simulink library "cyclopsLib"  (R2020a)
settings: Solver=VariableStepAuto  StartTime=0.0  StopTime=10.0  RelTol=1e-3
values from neighbouring files (symbols this model uses):
  agc_delay_lag = 32    [rev0BB_setup.m]
  agc_detector_coef = ones(1,agc_detector_taps)./agc_detector_taps    [rev0BB_setup.m]
  agc_sat_low = -agcSaturation    (= -12)    [rev0BB_setup.m]
  agc_sat_up = agcSaturation    (= 12)    [rev0BB_setup.m]
  agcDesired = 0    [rev0BB_setup.m]
  agcExpDomain = agcSaturation    (= 12)    [rev0BB_setup.m]
  agcExpResolution = 2^-3    (= 0.125)    [rev0BB_setup.m]
  agcPwrAvgNum = 128    [rev0BB_setup.m]
  agcSettleThresh = 0.65    [rev0BB_setup.m]
  agcStep = 2^-8    (= 0.00390625)    [rev0BB_setup.m]
  atanDomain = 5    [rev0BB_setup.m]
  atanResolution = 2^-9    (= 0.001953125)    [rev0BB_setup.m]
  bitsPerSymbolHeader = log2(radixHeader)    [rev0BB_setup.m]
  bitsPerSymbolMax = log2(radixMax)    [rev0BB_setup.m]
  cefEarlyWarning = 256    [rev0BB_setup.m]
  cefLen = length(x_CEF)    [rev0BB_setup.m]
  coarseCFOAdaptDelay = 1    [rev0BB_setup.m]
  cr_i = 0.020    (= 0.02)    [rev0BB_setup.m]
  cr_i_preamp = 2^-9    (= 0.001953125)    [rev0BB_setup.m]
  cr_int1_sat_low = -cr_integrator1_saturation    (= -0.6)    [rev0BB_setup.m]
  cr_int1_sat_up = cr_integrator1_saturation    (= 0.6)    [rev0BB_setup.m]
  cr_integrator1_decay = 1    [rev0BB_setup.m]
  cr_integrator1_saturation = 0.6    [rev0BB_setup.m]
  cr_mult_pipeline = 1    [rev0BB_setup.m]
  cr_p = 0.015    [rev0BB_setup.m]
  cr_sat2_low = -cr_saturation2    (= -0.6)    [rev0BB_setup.m]
  cr_sat2_up = cr_saturation2    (= 0.6)    [rev0BB_setup.m]
  cr_smooth_num = (1/cr_smooth_samples).*ones(1, cr_smooth_samples)    [rev0BB_setup.m]
  D_32 = [ 1,  4,  8,  2, 16]    [golay.m]    (also in rev0BB_setup.m)
  dataLenSymbols = header_len_bytes*8/bitsPerSymbolHeader + frame_len_bytes*8/bitsPerSymbol    [rev0BB_setup.m]
  delayToOutputFromDataFSM = lmsEqDepth/2-1 + regular_pipeline*9 + cr_mult_pipeline*4    (= 31)    [rev0BB_setup.m]
  enableTRFreqCorrection = true    [rev0BB_setup.m]
  expDomain = 3.3    [rev0BB_setup.m]
  expResolution = 2^-5    (= 0.03125)    [rev0BB_setup.m]
  expTol = .1    (= 0.1)    [rev0BB_setup.m]
  forceSlowRxStrobed = false    [rev0BB_setup.m]
  frac_lut_domain_cr = 64    [rev0BB_setup.m]
  frac_lut_range_max_coarse_cfo = 127    [rev0BB_setup.m]
  frac_lut_range_max_cr = 127    [rev0BB_setup.m]
  frac_lut_range_min_coarse_cfo = -frac_lut_range_max_coarse_cfo    (= -127)    [rev0BB_setup.m]
  frac_lut_range_min_cr = -frac_lut_range_max_cr    (= -127)    [rev0BB_setup.m]
  frac_lut_table_breaks_coarse_cfo = -frac_lut_domain_coarse_cfo:frac_lut_res_coarse_cfo:(frac_lut_domain_coarse_cfo-1)    [rev0BB_setup.m]
  frac_lut_table_breaks_cr = -frac_lut_domain_cr:frac_lut_res_cr:(frac_lut_domain_cr-1)    [rev0BB_setup.m]
  frac_lut_table_data_coarse_cfo = 1./frac_lut_table_breaks_coarse_cfo    [rev0BB_setup.m]
  frac_lut_table_data_cr = 1./frac_lut_table_breaks_cr    [rev0BB_setup.m]
  golay_type = 32    [rev0BB_setup.m]
  header_len_bytes = 8    [rev0BB_setup.m]
  lmsEqDepth = 38    [rev0BB_setup.m]
  lmsStep_init = 0.012    [rev0BB_setup.m]
  lmsStep_meta = (lmsStep_final - lmsStep_init)/cefLen    [rev0BB_setup.m]
  lnDomain = 16    [rev0BB_setup.m]
  lnResolution = 2^-3    (= 0.125)    [rev0BB_setup.m]
  minSTFPeaks = 3    [rev0BB_setup.m]
  mod_scheme_len_bytes = 1    [rev0BB_setup.m]
  modBPS = [1, 2, 4]    [rev0BB_setup.m]
  modKeys = [0, 1, 2]    [rev0BB_setup.m]
  mult_pipeline = 1    [rev0BB_setup.m]
  overSample = 4    [berCurve.m]    (also in rev0BB_setup.m)
  overSamplePer = 1/overSampleFreq    (= 1.25e-08)    [rev0BB_setup.m]
  qam16_demod_scale_factor = qam16_hdl_distance/qam16_power_normalized_distance    [rev0BB_setup.m]
  rcRxFilt = rcSqrtFilt    [rev0BB_setup.m]
  rcTxFilt = rcSqrtFilt    [rev0BB_setup.m]
  regular_pipeline = 1    [rev0BB_setup.m]
  rx_gain = 1    [rev0BB_setup.m]
  rx_gain_i = 1    [rev0BB_setup.m]
  rx_gain_q = 1    [rev0BB_setup.m]
  RxFeedbackPipelining = 128*3    (= 384)    [rev0BB_setup.m]
  stfLen = length(x_STF)    [rev0BB_setup.m]
  timing_differentiator_grpDelay_roundUp = ceil((timing_differentiator_len)/2)    [rev0BB_setup.m]
  timing_integrator1_decay = 0.999    [rev0BB_setup.m]
  timing_p = -1/2^2 -1/2^3    (= -0.375)    [rev0BB_setup.m]
  timing_tolerance = 4    [rev0BB_setup.m]
  timingRecoveryDoneSamplesEarly = 1    [rev0BB_setup.m]
  timingRecoveryDoneSamplesEarlyExtraDelay = -timingRecoveryDoneSamplesEarly+1    (= 0)    [rev0BB_setup.m]
  tr_int1_sat_low = -timing_integrate1_saturate    (= -0.0025)    [rev0BB_setup.m]
  tr_int1_sat_up = timing_integrate1_saturate    (= 0.0025)    [rev0BB_setup.m]
  tr_sat2_low = -timing_saturate2    (= -0.005)    [rev0BB_setup.m]
  tr_sat2_up = timing_saturate2    (= 0.005)    [rev0BB_setup.m]
  trigger = 0.40    (= 0.4)    [rev0BB_setup.m]
  trigger_tolerance = 0.35    [rev0BB_setup.m]
  W_32 = [-1,  1, -1,  1, -1]    [golay.m]    (also in rev0BB_setup.m)
  x_STFRepCount = nSpectrum_STFRepCount_short    (= 60)    [rev0BB_setup.m]
undefined symbols (not defined in the file or in its folder): agc_on, cr_integrator2_saturation, Fast_Rx_Partition, Fast_Slim_Rx_Partition, Feedback_Pipeline, freeze_en_agc, freeze_en_cr_int1, freeze_en_cr_int2, freeze_en_cr_phase, freeze_en_tr_int1, freeze_en_tr_int2, freeze_en_tr_phase, freeze_on_cef_done, freeze_on_stf_done, freeze_on_valid, i, post_cr_i_offset, post_cr_q_offset, rx_offset_correction_i, rx_offset_correction_q, Slow_Rx_Partition, timing_i, timing_i_pre_scale
libraries: simulink x62, helperLib x48, golayLib x15, commdigbbndpm3 x8, commdigbbndam3 x4, commfilt2 x3, hdlsllib x2, dspfdesign x1, simulink_need_slupdate x1, dspsigops x1, dsphdlsigops x1, $bdroot x1
(part 1 of 5)
settings Model: Creator=cyarp  LastModifiedBy=cyarp

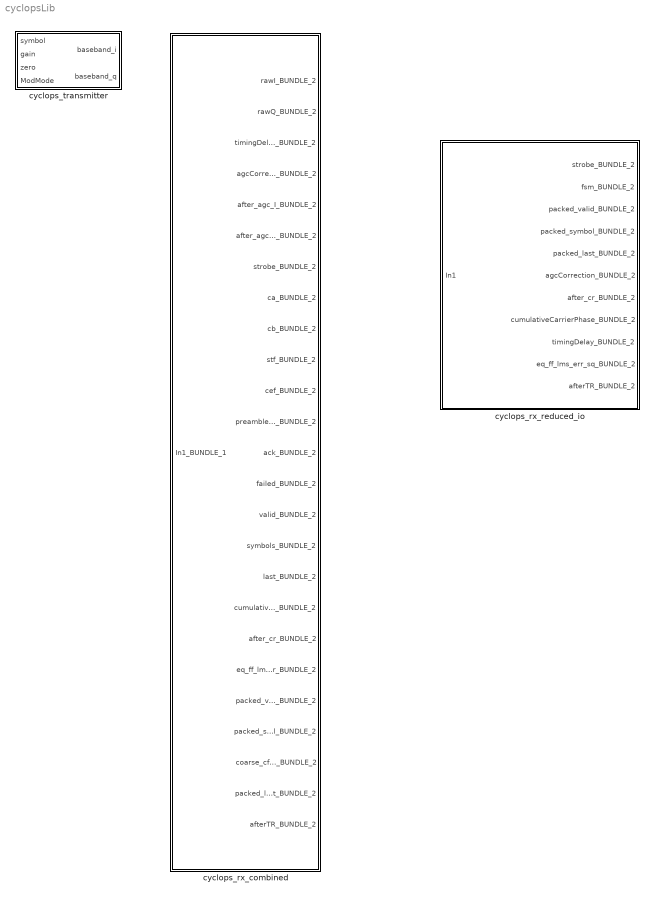
== system cyclopsLib ==
  cyclops_rx_combined : Subsystem  mask(Cyclops Rx){Fast_Slim_Rx_Partition=Fast_Slim_Rx_Partition, Fast_Rx_Partition=Fast_Rx_Partition, Slow_Rx_Partition=Slow_Rx_Partition, Feedback_Pipeline=Feedback_Pipeline}
      mask help: The Cyclops Rx with parameters for partitioning
  cyclops_rx_reduced_io : Subsystem  mask(Cyclops Rx (Reduced I/O)){Fast_Slim_Rx_Partition=1, Fast_Rx_Partition=2, Slow_Rx_Partition=2, Feedback_Pipeline=RxFeedbackPipelining}
      mask help: The Cyclops Rx with parameters for partitioning and reduced I/O
  cyclops_transmitter : Subsystem  mask(Cyclops Transmitter){Tx_Partition=1}
      mask help: The single channel transmitter for Cyclops. Parameterized with partition numbers

== system cyclopsLib/cyclops_rx_combined ==
  note: This feedback delay path is not latency critical.
      | Further pripelining should be OK
  In1_BUNDLE_1 : Inport
  fast_rx : Subsystem  TreatAsAtomicUnit=on
  slow_rx_encapsulated : Subsystem
  rawI_BUNDLE_2 : Outport  VectorParamsAs1DForOutWhenUnconnected=off
  rawQ_BUNDLE_2 : Outport  Port=2  VectorParamsAs1DForOutWhenUnconnected=off
  timingDelay_BUNDLE_2 : Outport  Port=3  VectorParamsAs1DForOutWhenUnconnected=off
  agcCorrection_BUNDLE_2 : Outport  Port=4  VectorParamsAs1DForOutWhenUnconnected=off
  after_agc_I_BUNDLE_2 : Outport  Port=5  VectorParamsAs1DForOutWhenUnconnected=off
  after_agc_Q_BUNDLE_2 : Outport  Port=6  VectorParamsAs1DForOutWhenUnconnected=off
  strobe_BUNDLE_2 : Outport  Port=7  VectorParamsAs1DForOutWhenUnconnected=off
  ca_BUNDLE_2 : Outport  Port=8  VectorParamsAs1DForOutWhenUnconnected=off
  cb_BUNDLE_2 : Outport  Port=9  VectorParamsAs1DForOutWhenUnconnected=off
  stf_BUNDLE_2 : Outport  Port=10  VectorParamsAs1DForOutWhenUnconnected=off
  cef_BUNDLE_2 : Outport  Port=11  VectorParamsAs1DForOutWhenUnconnected=off
  preambleDone_upsample_BUNDLE_2 : Outport  Port=12  VectorParamsAs1DForOutWhenUnconnected=off
  ack_BUNDLE_2 : Outport  Port=13  VectorParamsAs1DForOutWhenUnconnected=off
  failed_BUNDLE_2 : Outport  Port=14  VectorParamsAs1DForOutWhenUnconnected=off
  valid_BUNDLE_2 : Outport  Port=15  VectorParamsAs1DForOutWhenUnconnected=off
  symbols_BUNDLE_2 : Outport  Port=16  VectorParamsAs1DForOutWhenUnconnected=off
  last_BUNDLE_2 : Outport  Port=17  VectorParamsAs1DForOutWhenUnconnected=off
  cumulativeCarrierPhase_BUNDLE_2 : Outport  Port=18  VectorParamsAs1DForOutWhenUnconnected=off
  after_cr_BUNDLE_2 : Outport  Port=19  VectorParamsAs1DForOutWhenUnconnected=off
  eq_ff_lms_err_BUNDLE_2 : Outport  Port=20  VectorParamsAs1DForOutWhenUnconnected=off
  packed_valid_BUNDLE_2 : Outport  Port=21  VectorParamsAs1DForOutWhenUnconnected=off
  packed_symbol_BUNDLE_2 : Outport  Port=22  VectorParamsAs1DForOutWhenUnconnected=off
  coarse_cfo_correct_steps_BUNDLE_2 : Outport  Port=23  VectorParamsAs1DForOutWhenUnconnected=off
  packed_last_BUNDLE_2 : Outport  Port=24  VectorParamsAs1DForOutWhenUnconnected=off
  afterTR_BUNDLE_2 : Outport  Port=25
  wires:
  slow_rx_encapsulated/21(afterTR) -> afterTR_BUNDLE_2/1
  slow_rx_encapsulated/20(packet_reset_feedback) -> fast_rx/3(packet_reset_feedback)
  In1_BUNDLE_1/1 -> fast_rx/1(In1)
  fast_rx/4(rawI) -> rawI_BUNDLE_2/1
  fast_rx/5(rawQ) -> rawQ_BUNDLE_2/1
  fast_rx/6(timingDelay) -> timingDelay_BUNDLE_2/1
  fast_rx/7(agcCorrection) -> agcCorrection_BUNDLE_2/1
  fast_rx/8(after_agc_I) -> after_agc_I_BUNDLE_2/1
  fast_rx/9(after_agc_Q) -> after_agc_Q_BUNDLE_2/1
  fast_rx/1(data_out) -> slow_rx_encapsulated/1(data_in)
  fast_rx/2(agcPwrEst) -> slow_rx_encapsulated/2(agc_pwr_est)
  fast_rx/3(push) -> slow_rx_encapsulated/3(enb)
  slow_rx_encapsulated/1(strobe) -> strobe_BUNDLE_2/1
  slow_rx_encapsulated/2(ca) -> ca_BUNDLE_2/1
  slow_rx_encapsulated/3(cb) -> cb_BUNDLE_2/1
  slow_rx_encapsulated/4(stf) -> stf_BUNDLE_2/1
  slow_rx_encapsulated/5(cef) -> cef_BUNDLE_2/1
  slow_rx_encapsulated/6(preambleDone_upsample) -> preambleDone_upsample_BUNDLE_2/1
  slow_rx_encapsulated/7(ack) -> ack_BUNDLE_2/1
  slow_rx_encapsulated/8(failed) -> failed_BUNDLE_2/1
  slow_rx_encapsulated/9(valid) -> valid_BUNDLE_2/1
  slow_rx_encapsulated/10(symbols) -> symbols_BUNDLE_2/1
  slow_rx_encapsulated/11(last) -> last_BUNDLE_2/1
  slow_rx_encapsulated/12(cumulativeCarrierPhase) -> cumulativeCarrierPhase_BUNDLE_2/1
  slow_rx_encapsulated/13(after_cr) -> after_cr_BUNDLE_2/1
  slow_rx_encapsulated/14(eq_ff_lms_err) -> eq_ff_lms_err_BUNDLE_2/1
  slow_rx_encapsulated/15(freeze_out_pipelined) -> fast_rx/2(freeze)
  slow_rx_encapsulated/16(packed_valid) -> packed_valid_BUNDLE_2/1
  slow_rx_encapsulated/17(packed_symbol) -> packed_symbol_BUNDLE_2/1
  slow_rx_encapsulated/18(coarse_cfo_correct_steps) -> coarse_cfo_correct_steps_BUNDLE_2/1
  slow_rx_encapsulated/19(packed_last) -> packed_last_BUNDLE_2/1

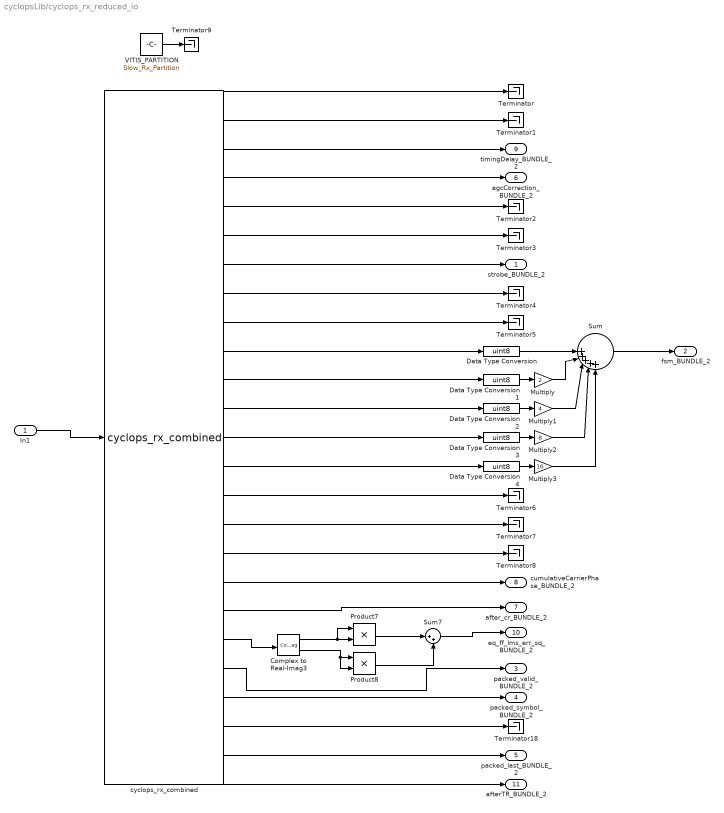
== system cyclopsLib/cyclops_rx_reduced_io ==
  In1 : Inport
  Complex to Real-Imag3 : ComplexToRealImag
  Data Type Conversion{,1..4} (5 alike) : DataTypeConversion  OutDataTypeStr=uint8
  Multiply : Gain  Gain=2  OutDataTypeStr=Inherit: Same as input
  Multiply1 : Gain  Gain=4  OutDataTypeStr=Inherit: Same as input
  Multiply2 : Gain  Gain=8  OutDataTypeStr=Inherit: Same as input
  Multiply3 : Gain  Gain=16  ParamDataTypeStr=Inherit: Same as input
  Product7 : Product
  Product8 : Product
  Sum : Sum  Inputs=||||+++++  OutDataTypeStr=Inherit: Same as first input
  Sum7 : Sum  Inputs=|++
  Terminator{,1..9,18} (11 alike) : Terminator
  VITIS_PARTITION : Constant  Value=Slow_Rx_Partition
  cyclops_rx_combined : $bdroot/cyclops_rx_combined  Fast_Slim_Rx_Partition=Fast_Slim_Rx_Partition  Fast_Rx_Partition=Fast_Rx_Partition  Slow_Rx_Partition=Slow_Rx_Partition  Feedback_Pipeline=Feedback_Pipeline
  strobe_BUNDLE_2 : Outport
  fsm_BUNDLE_2 : Outport  Port=2
  packed_valid_BUNDLE_2 : Outport  Port=3
  packed_symbol_BUNDLE_2 : Outport  Port=4
  packed_last_BUNDLE_2 : Outport  Port=5
  agcCorrection_BUNDLE_2 : Outport  Port=6
  after_cr_BUNDLE_2 : Outport  Port=7
  cumulativeCarrierPhase_BUNDLE_2 : Outport  Port=8
  timingDelay_BUNDLE_2 : Outport  Port=9
  eq_ff_lms_err_sq_BUNDLE_2 : Outport  Port=10
  afterTR_BUNDLE_2 : Outport  Port=11
  wires:
  cyclops_rx_combined/25 -> afterTR_BUNDLE_2/1
  cyclops_rx_combined/18 -> cumulativeCarrierPhase_BUNDLE_2/1
  In1/1 -> cyclops_rx_combined/1
  cyclops_rx_combined/3 -> timingDelay_BUNDLE_2/1
  cyclops_rx_combined/24 -> packed_last_BUNDLE_2/1
  cyclops_rx_combined/9 -> Terminator5/1
  cyclops_rx_combined/12 -> Data Type Conversion2/1
  cyclops_rx_combined/5 -> Terminator2/1
  cyclops_rx_combined/21 -> packed_valid_BUNDLE_2/1
  Complex to Real-Imag3/1 -> Product7/1, Product7/2
  Data Type Conversion4/1 -> Multiply3/1
  cyclops_rx_combined/17 -> Terminator8/1
  cyclops_rx_combined/16 -> Terminator7/1
  cyclops_rx_combined/10 -> Data Type Conversion/1
  cyclops_rx_combined/14 -> Data Type Conversion4/1
  Multiply2/1 -> Sum/4
  cyclops_rx_combined/8 -> Terminator4/1
  cyclops_rx_combined/4 -> agcCorrection_BUNDLE_2/1
  Multiply3/1 -> Sum/5
  cyclops_rx_combined/23 -> Terminator18/1
  cyclops_rx_combined/19 -> after_cr_BUNDLE_2/1
  cyclops_rx_combined/2 -> Terminator1/1
  Sum7/1 -> eq_ff_lms_err_sq_BUNDLE_2/1
  Multiply1/1 -> Sum/3
  Product8/1 -> Sum7/2
  Data Type Conversion3/1 -> Multiply2/1
  Multiply/1 -> Sum/2
  Complex to Real-Imag3/2 -> Product8/2, Product8/1
  cyclops_rx_combined/11 -> Data Type Conversion1/1
  cyclops_rx_combined/6 -> Terminator3/1
  Sum/1 -> fsm_BUNDLE_2/1
  cyclops_rx_combined/13 -> Data Type Conversion3/1
  Product7/1 -> Sum7/1
  Data Type Conversion1/1 -> Multiply/1
  cyclops_rx_combined/20 -> Complex to Real-Imag3/1
  Data Type Conversion/1 -> Sum/1
  Data Type Conversion2/1 -> Multiply1/1
  cyclops_rx_combined/1 -> Terminator/1
  cyclops_rx_combined/15 -> Terminator6/1
  cyclops_rx_combined/7 -> strobe_BUNDLE_2/1
  cyclops_rx_combined/22 -> packed_symbol_BUNDLE_2/1
  VITIS_PARTITION/1 -> Terminator9/1

== system cyclopsLib/cyclops_transmitter ==
  note: Logic for zero filling in upsample
  symbol : Inport  SampleTime=overSamplePer
  gain : Inport  Port=2  SampleTime=overSamplePer
  zero : Inport  Port=3  OutDataTypeStr=boolean  SampleTime=overSamplePer
  ModMode : Inport  Port=4  SampleTime=overSamplePer
  Compare To Zero : simulink/Logic and Bit Operations/Compare To Zero  relop=~=  OutDataTypeStr=boolean
  Constant : Constant  Value=0  OutDataTypeStr=Inherit: Inherit via back propagation  SampleTime=-1
  Constant1 : Constant  Value=0  OutDataTypeStr=Inherit: Inherit via back propagation  SampleTime=-1
  Logical Operator : Logic  Operator=OR  AllPortsSameDT=off  OutDataTypeStr=boolean
  Real-Imag to Complex : RealImagToComplex
  Switch : Switch
  Terminator2 : Terminator
  VITIS_PARTITION : Constant  Value=Tx_Partition
  modulator : Subsystem
  part2_noLPF : Subsystem
  pipeline_delay1 : Delay  DelayLength=regular_pipeline
  raised_cosine : Subsystem
  zero_fill_counter : Subsystem
  baseband_i : Outport  SampleTime=overSamplePer  InitialOutput=[0]  VectorParamsAs1DForOutWhenUnconnected=off
  baseband_q : Outport  Port=2  SampleTime=overSamplePer  InitialOutput=[0]  VectorParamsAs1DForOutWhenUnconnected=off
  wires:
  pipeline_delay1/1 -> raised_cosine/1(In1)
  zero/1 -> Logical Operator/1
  Constant1/1 -> Real-Imag to Complex/2
  Constant/1 -> Real-Imag to Complex/1
  Real-Imag to Complex/1 -> Switch/1
  Logical Operator/1 -> Switch/2
  Compare To Zero/1 -> Logical Operator/2
  zero_fill_counter/1(Out1) -> Compare To Zero/1
  Switch/1 -> pipeline_delay1/1
  ModMode/1 -> modulator/1(mod_mode)
  symbol/1 -> modulator/2(symbol)
  modulator/1(point) -> Switch/3
  VITIS_PARTITION/1 -> Terminator2/1
  gain/1 -> part2_noLPF/1(Gain)
  raised_cosine/1(Out1) -> part2_noLPF/2(In)
  part2_noLPF/1(I) -> baseband_i/1
  part2_noLPF/2(Q) -> baseband_q/1

== system cyclopsLib/cyclops_rx_combined/fast_rx ==
  In1 : Inport
  freeze : Inport  Port=2
  packet_reset_feedback : Inport  Port=3
  fast_rx_baseband_encapsulated : Subsystem
  fast_rx_baseband_slim_encapsulated : Subsystem
  data_out : Outport  VectorParamsAs1DForOutWhenUnconnected=off
  agcPwrEst : Outport  Port=2  VectorParamsAs1DForOutWhenUnconnected=off
  push : Outport  Port=3  VectorParamsAs1DForOutWhenUnconnected=off
  rawI : Outport  Port=4  VectorParamsAs1DForOutWhenUnconnected=off
  rawQ : Outport  Port=5  VectorParamsAs1DForOutWhenUnconnected=off
  timingDelay : Outport  Port=6  VectorParamsAs1DForOutWhenUnconnected=off
  agcCorrection : Outport  Port=7  VectorParamsAs1DForOutWhenUnconnected=off
  after_agc_I : Outport  Port=8  VectorParamsAs1DForOutWhenUnconnected=off
  after_agc_Q : Outport  Port=9  VectorParamsAs1DForOutWhenUnconnected=off
  wires:
  packet_reset_feedback/1 -> fast_rx_baseband_encapsulated/3(packet_reset_feedback)
  freeze/1 -> fast_rx_baseband_slim_encapsulated/2(agc_freeze)
  fast_rx_baseband_slim_encapsulated/3(rawI) -> rawI/1
  fast_rx_baseband_slim_encapsulated/4(rawQ) -> rawQ/1
  fast_rx_baseband_slim_encapsulated/5(agcPwrEst) -> agcPwrEst/1
  fast_rx_baseband_slim_encapsulated/6(agcCorrection) -> agcCorrection/1
  fast_rx_baseband_encapsulated/2(data_out) -> data_out/1
  fast_rx_baseband_encapsulated/1(push) -> push/1
  fast_rx_baseband_encapsulated/5(after_agc_Q) -> after_agc_Q/1
  fast_rx_baseband_encapsulated/3(timing_delay) -> timingDelay/1
  fast_rx_baseband_encapsulated/4(after_agc_I) -> after_agc_I/1
  fast_rx_baseband_slim_encapsulated/1(sig_out_i) -> fast_rx_baseband_encapsulated/1(sig_in_i)
  fast_rx_baseband_slim_encapsulated/2(sig_out_q) -> fast_rx_baseband_encapsulated/2(sig_in_q)
  In1/1 -> fast_rx_baseband_slim_encapsulated/1(baseband_in)

== system cyclopsLib/cyclops_rx_combined/slow_rx_encapsulated ==
  note: This feedback delay path is not latency critical.
      | Further pripelining should be OK
  data_in : Inport
  agc_pwr_est : Inport  Port=2
  enb : Inport  Port=3
  Delay1 : Delay  Commented=on  DelayLength=128  InitialCondition=false
  Terminator : Terminator
  VITIS_PARTITION : Constant  Value=Slow_Rx_Partition
  slow_rx : Subsystem  TreatAsAtomicUnit=on
  strobe : Outport  VectorParamsAs1DForOutWhenUnconnected=off
  ca : Outport  Port=2  VectorParamsAs1DForOutWhenUnconnected=off
  cb : Outport  Port=3  VectorParamsAs1DForOutWhenUnconnected=off
  stf : Outport  Port=4  VectorParamsAs1DForOutWhenUnconnected=off
  cef : Outport  Port=5  VectorParamsAs1DForOutWhenUnconnected=off
  preambleDone_upsample : Outport  Port=6  VectorParamsAs1DForOutWhenUnconnected=off
  ack : Outport  Port=7  VectorParamsAs1DForOutWhenUnconnected=off
  failed : Outport  Port=8  VectorParamsAs1DForOutWhenUnconnected=off
  valid : Outport  Port=9  VectorParamsAs1DForOutWhenUnconnected=off
  symbols : Outport  Port=10  VectorParamsAs1DForOutWhenUnconnected=off
  last : Outport  Port=11  VectorParamsAs1DForOutWhenUnconnected=off
  cumulativeCarrierPhase : Outport  Port=12  VectorParamsAs1DForOutWhenUnconnected=off
  after_cr : Outport  Port=13  VectorParamsAs1DForOutWhenUnconnected=off
  eq_ff_lms_err : Outport  Port=14  VectorParamsAs1DForOutWhenUnconnected=off
  freeze_out_pipelined : Outport  Port=15  VectorParamsAs1DForOutWhenUnconnected=off
  packed_valid : Outport  Port=16  VectorParamsAs1DForOutWhenUnconnected=off
  packed_symbol : Outport  Port=17  VectorParamsAs1DForOutWhenUnconnected=off
  coarse_cfo_correct_steps : Outport  Port=18  VectorParamsAs1DForOutWhenUnconnected=off
  packed_last : Outport  Port=19  VectorParamsAs1DForOutWhenUnconnected=off
  packet_reset_feedback : Outport  Port=20
  afterTR : Outport  Port=21
  wires:
  slow_rx/21(afterTR) -> afterTR/1
  slow_rx/20(packet_reset_feedback) -> packet_reset_feedback/1
  slow_rx/11(last) -> last/1
  slow_rx/12(cumulativeCarrierPhase) -> cumulativeCarrierPhase/1
  slow_rx/8(failed) -> failed/1
  slow_rx/16(packed_symbol) -> packed_symbol/1
  slow_rx/15(packed_valid) -> packed_valid/1
  slow_rx/13(after_cr) -> after_cr/1
  slow_rx/14(eq_ff_lms_err) -> eq_ff_lms_err/1
  data_in/1 -> slow_rx/1(data_in)
  slow_rx/6(preambleDone_upsample) -> preambleDone_upsample/1
  agc_pwr_est/1 -> slow_rx/2(agc_pwr_est)
  enb/1 -> slow_rx/3(enb)
  slow_rx/1(strobe) -> strobe/1
  slow_rx/2(ca) -> ca/1
  slow_rx/3(cb) -> cb/1
  slow_rx/4(stf) -> stf/1
  slow_rx/5(cef) -> cef/1
  slow_rx/7(ack) -> ack/1
  slow_rx/10(symbols) -> symbols/1
  slow_rx/9(valid) -> valid/1
  VITIS_PARTITION/1 -> Terminator/1
  slow_rx/17(freeze_out) -> freeze_out_pipelined/1
  slow_rx/18(coarse_cfo_correct_steps) -> coarse_cfo_correct_steps/1
  slow_rx/19(packed_last) -> packed_last/1

== system cyclopsLib/cyclops_transmitter/modulator ==
  mod_mode : Inport
  symbol : Inport  Port=2
  BPSK Modulator Baseband : commdigbbndpm3/BPSK Modulator Baseband  Ph=0  outDtype=single  outWordLen=16  outUDDataType=sfix(16)  outFracLenMode=User-defined  outFracLen=13  outDataTypeStr=single  outLastDataTypeStr=single
  Bitwise Operator : simulink/Logic and Bit Operations/Bitwise Operator  logicop=AND  UseBitMask=off  NumInputPorts=2  BitMask=bin2dec('11011001')  BitMaskRealWorld=Stored Integer
  Bitwise Operator1 : simulink/Logic and Bit Operations/Bitwise Operator  logicop=AND  UseBitMask=off  NumInputPorts=2  BitMask=bin2dec('11011001')  BitMaskRealWorld=Stored Integer
  Bitwise Operator2 : simulink/Logic and Bit Operations/Bitwise Operator  logicop=AND  UseBitMask=off  NumInputPorts=2  BitMask=bin2dec('11011001')  BitMaskRealWorld=Stored Integer
  Constant : Constant  Value=bin2dec('000001')  OutDataTypeStr=Inherit: Inherit via back propagation
  Constant1 : Constant  Value=bin2dec('000011')  OutDataTypeStr=Inherit: Inherit via back propagation
  Constant2 : Constant  OutDataTypeStr=Inherit: Inherit via back propagation  SampleTime=-1
  Constant3 : Constant  Value=bin2dec('001111')  OutDataTypeStr=Inherit: Inherit via back propagation
  Data Type Conversion : DataTypeConversion  OutDataTypeStr=uint32
  Data Type Conversion1 : DataTypeConversion  OutDataTypeStr=uint32
  Data Type Conversion2 : DataTypeConversion  OutDataTypeStr=uint32
  Data Type Conversion3 : DataTypeConversion  Commented=on  OutDataTypeStr=fixdt(0,1,0)
  Data Type Conversion4 : DataTypeConversion  Commented=on  OutDataTypeStr=fixdt(0,2,0)
  Data Type Conversion5 : DataTypeConversion  Commented=on  OutDataTypeStr=fixdt(0,4,0)
  Extract Bits : simulink/Logic and Bit Operations/Extract Bits  Commented=on  bitsToExtract=Range of bits  numBits=8  bitIdxRange=[0 0]  outScalingMode=Preserve fixed-point scaling
  Extract Bits1 : simulink/Logic and Bit Operations/Extract Bits  Commented=on  bitsToExtract=Range of bits  numBits=8  bitIdxRange=[0 1]  outScalingMode=Preserve fixed-point scaling
  Extract Bits2 : simulink/Logic and Bit Operations/Extract Bits  Commented=on  bitsToExtract=Range of bits  numBits=8  bitIdxRange=[0 3]  outScalingMode=Preserve fixed-point scaling
  Multiport Switch : MultiPortSwitch
  QPSK Modulator Baseband : commdigbbndpm3/QPSK Modulator Baseband  InType=Integer  Enc=Gray  Ph=pi/4  outDtype=single  outWordLen=16  outUDDataType=sfix(16)  outFracLenMode=User-defined  outFracLen=13  outDataTypeStr=single  outLastDataTypeStr=single
  Rectangular QAM Modulator Baseband : commdigbbndam3/Rectangular QAM Modulator Baseband  M=16  InType=Integer  Enc=Gray  Mapping=[0:15]  PowType=Average Power  MinDist=2  AvgPow=1  PeakPow=1  Ph=0  outDtype=single  outWordLen=16  outUDDataType=sfix(16)  outFracLenMode=User-defined  outFracLen=13  outDataTypeStr=single  outLastDataTypeStr=single
  Sum : Sum  Inputs=|++  OutDataTypeStr=Inherit: Same as first input
  point : Outport  VectorParamsAs1DForOutWhenUnconnected=off
  wires:
  Multiport Switch/1 -> point/1
  BPSK Modulator Baseband/1 -> Multiport Switch/2
  Rectangular QAM Modulator Baseband/1 -> Multiport Switch/4
  Data Type Conversion/1 -> BPSK Modulator Baseband/1
  QPSK Modulator Baseband/1 -> Multiport Switch/3
  symbol/1 -> Bitwise Operator/1, Bitwise Operator2/1, Bitwise Operator1/1
  mod_mode/1 -> Sum/1
  Sum/1 -> Multiport Switch/1
  Constant2/1 -> Sum/2
  Data Type Conversion1/1 -> QPSK Modulator Baseband/1
  Data Type Conversion2/1 -> Rectangular QAM Modulator Baseband/1
  Bitwise Operator/1 -> Data Type Conversion/1
  Bitwise Operator1/1 -> Data Type Conversion1/1
  Bitwise Operator2/1 -> Data Type Conversion2/1
  Constant/1 -> Bitwise Operator/2
  Constant1/1 -> Bitwise Operator1/2
  Constant3/1 -> Bitwise Operator2/2

== system cyclopsLib/cyclops_transmitter/part2_noLPF ==
  Gain : Inport
  In : Inport  Port=2
  Complex to Real-Imag : ComplexToRealImag
  Gain1 : Gain  Gain=2  OutDataTypeStr=Inherit: Same as input
  Product : Product  OutDataTypeStr=Inherit: Same as first input
  mult_delay1 : Delay  DelayLength=mult_pipeline
  mult_delay2 : Delay  DelayLength=mult_pipeline
  pipeline_delay3 : Delay  DelayLength=regular_pipeline
  I : Outport
  Q : Outport  Port=2
  wires:
  Complex to Real-Imag/1 -> I/1
  Gain/1 -> mult_delay1/1
  In/1 -> Gain1/1
  Complex to Real-Imag/2 -> Q/1
  Product/1 -> pipeline_delay3/1
  pipeline_delay3/1 -> Complex to Real-Imag/1
  Gain1/1 -> mult_delay2/1
  mult_delay1/1 -> Product/2
  mult_delay2/1 -> Product/1

== system cyclopsLib/cyclops_transmitter/raised_cosine ==
  note: (a+bj)(c+dj) = ac+adj+bcj-bd
      | If d = 0 | = ac + bcj
  note: Raised Cosine Filter Can be Split because it is Real (use 2 multiplies instead of 4 per tap)
  note: Note: the tool should optomize a single FIR filter to this config due to 0 propogation. However, will make explicit for now
  In1 : Inport
  Discrete FIR Filter : DiscreteFir  FilterStructure=Direct form transposed  Coefficients=rcTxFilt
  Raised Cosine Transmit Filter : commfilt2/Raised Cosine Transmit Filter  Commented=on  filtType=Square root  R=.1  filtSpan=16  N=4  filterGain=1  RateOptions=Allow multirate processing  framing=Mute  checkCoeff=on  variableName=rcTxFilt  checkGain=Normalized  sampMode=Mute  saveAsFlag=0  currentFiltSpan=16  D=(16)/2  launchFVT=on  roundingMode=Floor  overflowMode=off  coeffDataTypeStr=Inherit: Same word length as input  coeffMin=[]  coeffMax=[]  coeffLastDataTypeStr=Inherit: Same word length as input  outputDataTypeStr=Inherit: Same as accumulator  outputMin=[]  outputMax=[]  outputLastDataTypeStr=Inherit: Same as accumulator
  Raised Cosine Transmit Filter_full : commfilt2/Raised Cosine Transmit Filter  Commented=on  filtType=Normal  R=0.08  filtSpan=40  N=4  filterGain=1  RateOptions=Allow multirate processing  framing=Mute  checkCoeff=on  variableName=rcTxFilt_full  checkGain=Normalized  sampMode=Mute  saveAsFlag=0  currentFiltSpan=40  D=(40)/2  launchFVT=on  roundingMode=Floor  overflowMode=off  coeffDataTypeStr=Inherit: Same word length as input  coeffMin=[]  coeffMax=[]  coeffLastDataTypeStr=Inherit: Same word length as input  outputDataTypeStr=Inherit: Same as accumulator  outputMin=[]  outputMax=[]  outputLastDataTypeStr=Inherit: Same as accumulator
  mult_delay : Delay  DelayLength=mult_pipeline
  mult_delay1 : Delay  DelayLength=mult_pipeline
  Out1 : Outport  VectorParamsAs1DForOutWhenUnconnected=off
  wires:
  In1/1 -> mult_delay/1
  mult_delay/1 -> Discrete FIR Filter/1
  mult_delay1/1 -> Out1/1
  Discrete FIR Filter/1 -> mult_delay1/1

== system cyclopsLib/cyclops_transmitter/zero_fill_counter ==
  Compare To Constant : simulink/Logic and Bit Operations/Compare To Constant  relop=>=  const=3  OutDataTypeStr=boolean
  Constant2 : Constant  OutDataTypeStr=uint8  SampleTime=-1
  Constant3 : Constant  Value=0  OutDataTypeStr=uint8  SampleTime=-1
  Delay : Delay  DelayLength=1  InitialCondition=0
  Sum : Sum  Inputs=|++  OutDataTypeStr=Inherit: Same as first input
  Switch1 : Switch  Criteria=u2 > Threshold
  Out1 : Outport  VectorParamsAs1DForOutWhenUnconnected=off
  wires:
  Switch1/1 -> Delay/1
  Compare To Constant/1 -> Switch1/2
  Constant3/1 -> Switch1/1
  Delay/1 -> Out1/1, Sum/2, Compare To Constant/1
  Constant2/1 -> Sum/1
  Sum/1 -> Switch1/3

== system cyclopsLib/cyclops_rx_combined/fast_rx/fast_rx_baseband_encapsulated ==
  sig_in_i : Inport
  sig_in_q : Inport  Port=2
  packet_reset_feedback : Inport  Port=3
  Delay1 : Delay  DelayLength=Feedback_Pipeline  InitialCondition=false
  Terminator : Terminator
  VITIS_PARTITION : Constant  Value=Fast_Rx_Partition
  fast_rx_baseband : Subsystem  TreatAsAtomicUnit=on
  freeze_en_tr_int1 : Constant  Commented=on  Value=freeze_en_tr_int1  OutDataTypeStr=Inherit: Inherit via back propagation  SampleTime=-1
  freeze_en_tr_int2 : Constant  Commented=on  Value=freeze_en_tr_int2  OutDataTypeStr=Inherit: Inherit via back propagation  SampleTime=-1
  freeze_en_tr_phase : Constant  Commented=on  Value=freeze_en_tr_phase  OutDataTypeStr=Inherit: Inherit via back propagation  SampleTime=-1
  timing_i : Constant  Commented=on  Value=timing_i  OutDataTypeStr=Inherit: Inherit via back propagation  SampleTime=-1
  timing_i_pre_scale : Constant  Commented=on  Value=timing_i_pre_scale  OutDataTypeStr=Inherit: Inherit via back propagation  SampleTime=-1
  timing_integrator1_decay : Constant  Commented=on  Value=timing_integrator1_decay  OutDataTypeStr=Inherit: Inherit via back propagation  SampleTime=-1
  timing_p : Constant  Value=timing_p  OutDataTypeStr=Inherit: Inherit via back propagation  SampleTime=-1
  tr_int1_sat_low : Constant  Commented=on  Value=tr_int1_sat_low  OutDataTypeStr=Inherit: Inherit via back propagation  SampleTime=-1
  tr_int1_sat_up : Constant  Commented=on  Value=tr_int1_sat_up  OutDataTypeStr=Inherit: Inherit via back propagation  SampleTime=-1
  tr_sat2_low1 : Constant  Commented=on  Value=tr_sat2_low  OutDataTypeStr=Inherit: Inherit via back propagation  SampleTime=-1
  tr_sat2_up1 : Constant  Commented=on  Value=tr_sat2_up  OutDataTypeStr=Inherit: Inherit via back propagation  SampleTime=-1
  push : Outport  VectorParamsAs1DForOutWhenUnconnected=off
  data_out : Outport  Port=2  VectorParamsAs1DForOutWhenUnconnected=off
  timing_delay : Outport  Port=3  VectorParamsAs1DForOutWhenUnconnected=off
  after_agc_I : Outport  Port=4  VectorParamsAs1DForOutWhenUnconnected=off
  after_agc_Q : Outport  Port=5  VectorParamsAs1DForOutWhenUnconnected=off
  wires:
  timing_p/1 -> fast_rx_baseband/3(timing_p)
  Delay1/1 -> fast_rx_baseband/4(packet_reset_feedback)
  packet_reset_feedback/1 -> Delay1/1
  fast_rx_baseband/3(timing_delay) -> timing_delay/1
  fast_rx_baseband/2(data_out) -> data_out/1
  fast_rx_baseband/1(push) -> push/1
  fast_rx_baseband/5(after_agc_Q) -> after_agc_Q/1
  fast_rx_baseband/4(after_agc_I) -> after_agc_I/1
  sig_in_i/1 -> fast_rx_baseband/1(sig_in_i)
  sig_in_q/1 -> fast_rx_baseband/2(sig_in_q)
  VITIS_PARTITION/1 -> Terminator/1

== system cyclopsLib/cyclops_rx_combined/fast_rx/fast_rx_baseband_slim_encapsulated ==
  baseband_in : Inport
  agc_freeze : Inport  Port=2
  Complex to Real-Imag : ComplexToRealImag
  Delay : Delay  DelayLength=Feedback_Pipeline  InitialCondition=false
  Terminator2 : Terminator
  VITIS_PARTITION : Constant  Value=Fast_Slim_Rx_Partition
  agcDesired : Constant  Value=agcDesired  OutDataTypeStr=Inherit: Inherit via back propagation  SampleTime=-1
  agcStepSize : Constant  Value=agcStep  OutDataTypeStr=Inherit: Inherit via back propagation  SampleTime=-1
  agc_on : Constant  Value=agc_on  OutDataTypeStr=Inherit: Inherit via back propagation  SampleTime=-1
  agc_sat_low : Constant  Value=agc_sat_low  OutDataTypeStr=Inherit: Inherit via back propagation  SampleTime=-1
  agc_sat_up : Constant  Value=agc_sat_up  OutDataTypeStr=Inherit: Inherit via back propagation  SampleTime=-1
  freeze_en_agc : Constant  Value=freeze_en_agc  OutDataTypeStr=Inherit: Inherit via back propagation  SampleTime=-1
  pre_gain_i : Constant  Value=rx_gain_i  OutDataTypeStr=Inherit: Inherit via back propagation  SampleTime=overSamplePer
  pre_gain_q : Constant  Value=rx_gain_q  OutDataTypeStr=Inherit: Inherit via back propagation  SampleTime=overSamplePer
  rx_gain : Constant  Value=rx_gain  OutDataTypeStr=Inherit: Inherit via back propagation  SampleTime=overSamplePer
  rx_offset_i : Constant  Value=rx_offset_correction_i  OutDataTypeStr=Inherit: Inherit via back propagation  SampleTime=overSamplePer
  rx_offset_q : Constant  Value=rx_offset_correction_q  OutDataTypeStr=Inherit: Inherit via back propagation  SampleTime=overSamplePer
  slim_fast_rx : Subsystem  TreatAsAtomicUnit=on
  sig_out_i : Outport  VectorParamsAs1DForOutWhenUnconnected=off
  sig_out_q : Outport  Port=2  VectorParamsAs1DForOutWhenUnconnected=off
  rawI : Outport  Port=3  VectorParamsAs1DForOutWhenUnconnected=off
  rawQ : Outport  Port=4  VectorParamsAs1DForOutWhenUnconnected=off
  agcPwrEst : Outport  Port=5  VectorParamsAs1DForOutWhenUnconnected=off
  agcCorrection : Outport  Port=6  VectorParamsAs1DForOutWhenUnconnected=off
  wires:
  slim_fast_rx/4(rawQ) -> rawQ/1
  agc_sat_up/1 -> slim_fast_rx/13(agc_sat_up)
  pre_gain_q/1 -> slim_fast_rx/4(pre_gain_q)
  rx_offset_i/1 -> slim_fast_rx/5(offset_i)
  freeze_en_agc/1 -> slim_fast_rx/12(freeze_en_agc)
  pre_gain_i/1 -> slim_fast_rx/3(pre_gain_i)
  agcDesired/1 -> slim_fast_rx/8(agc_desired)
  agc_sat_low/1 -> slim_fast_rx/14(agc_sat_low)
  Complex to Real-Imag/1 -> slim_fast_rx/1(baseband_i)
  baseband_in/1 -> Complex to Real-Imag/1
  agcStepSize/1 -> slim_fast_rx/9(agc_step_size)
  slim_fast_rx/1(sig_out_i) -> sig_out_i/1
  agc_on/1 -> slim_fast_rx/10(agc_on)
  slim_fast_rx/5(agcPwrEst) -> agcPwrEst/1
  rx_offset_q/1 -> slim_fast_rx/6(offset_q)
  rx_gain/1 -> slim_fast_rx/7(gain)
  slim_fast_rx/2(sig_out_q) -> sig_out_q/1
  slim_fast_rx/6(agcCorrection) -> agcCorrection/1
  slim_fast_rx/3(rawI) -> rawI/1
  Complex to Real-Imag/2 -> slim_fast_rx/2(baseband_q)
  VITIS_PARTITION/1 -> Terminator2/1
  agc_freeze/1 -> Delay/1
  Delay/1 -> slim_fast_rx/11(agc_freeze)

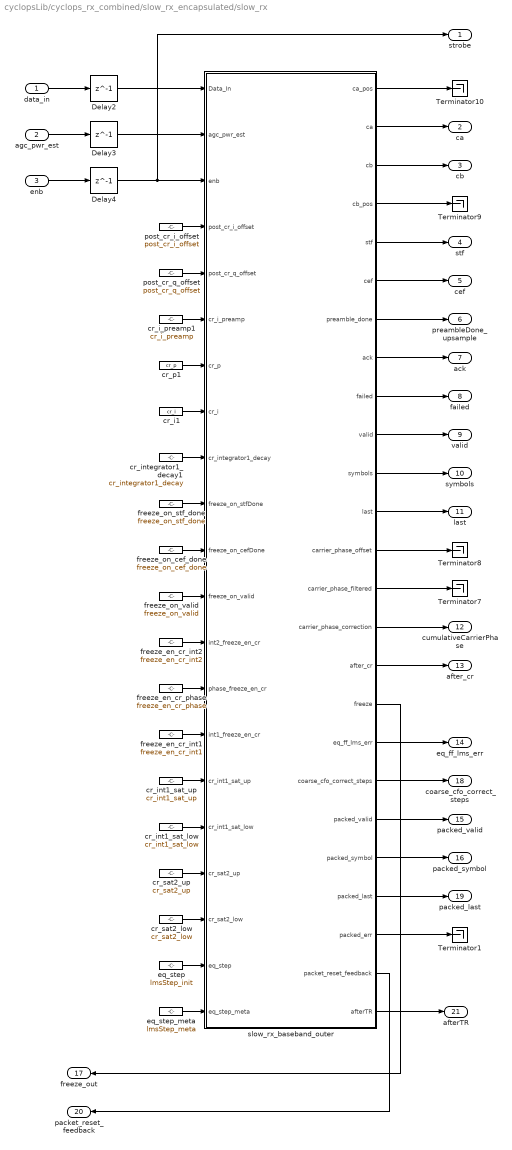
== system cyclopsLib/cyclops_rx_combined/slow_rx_encapsulated/slow_rx ==
  data_in : Inport
  agc_pwr_est : Inport  Port=2
  enb : Inport  Port=3
  Delay2 : Delay  DelayLength=1
  Delay3 : Delay  DelayLength=1
  Delay4 : Delay  DelayLength=1
  Terminator{1,7..10} (5 alike) : Terminator
  cr_i1 : Constant  Value=cr_i  OutDataTypeStr=Inherit: Inherit via back propagation  SampleTime=-1
  cr_i_preamp1 : Constant  Value=cr_i_preamp  OutDataTypeStr=Inherit: Inherit via back propagation  SampleTime=-1
  cr_int1_sat_low : Constant  Value=cr_int1_sat_low  OutDataTypeStr=Inherit: Inherit via back propagation  SampleTime=-1
  cr_int1_sat_up : Constant  Value=cr_int1_sat_up  OutDataTypeStr=Inherit: Inherit via back propagation  SampleTime=-1
  cr_integrator1_decay1 : Constant  Value=cr_integrator1_decay  OutDataTypeStr=Inherit: Inherit via back propagation  SampleTime=-1
  cr_p1 : Constant  Value=cr_p  OutDataTypeStr=Inherit: Inherit via back propagation  SampleTime=-1
  cr_sat2_low : Constant  Value=cr_sat2_low  OutDataTypeStr=Inherit: Inherit via back propagation  SampleTime=-1
  cr_sat2_up : Constant  Value=cr_sat2_up  OutDataTypeStr=Inherit: Inherit via back propagation  SampleTime=-1
  eq_step : Constant  Value=lmsStep_init  OutDataTypeStr=Inherit: Inherit via back propagation  SampleTime=-1
  eq_step_meta : Constant  Value=lmsStep_meta  OutDataTypeStr=Inherit: Inherit via back propagation  SampleTime=-1
  freeze_en_cr_int1 : Constant  Value=freeze_en_cr_int1  OutDataTypeStr=Inherit: Inherit via back propagation  SampleTime=-1
  freeze_en_cr_int2 : Constant  Value=freeze_en_cr_int2  OutDataTypeStr=Inherit: Inherit via back propagation  SampleTime=-1
  freeze_en_cr_phase : Constant  Value=freeze_en_cr_phase  OutDataTypeStr=Inherit: Inherit via back propagation  SampleTime=-1
  freeze_on_cef_done : Constant  Value=freeze_on_cef_done  OutDataTypeStr=Inherit: Inherit via back propagation  SampleTime=-1
  freeze_on_stf_done : Constant  Value=freeze_on_stf_done  OutDataTypeStr=Inherit: Inherit via back propagation  SampleTime=-1
  freeze_on_valid : Constant  Value=freeze_on_valid  OutDataTypeStr=Inherit: Inherit via back propagation  SampleTime=-1
  post_cr_i_offset : Constant  Value=post_cr_i_offset  OutDataTypeStr=Inherit: Inherit via back propagation  SampleTime=-1
  post_cr_q_offset : Constant  Value=post_cr_q_offset  OutDataTypeStr=Inherit: Inherit via back propagation  SampleTime=-1
  slow_rx_baseband_outer : Subsystem  TreatAsAtomicUnit=on
  strobe : Outport  VectorParamsAs1DForOutWhenUnconnected=off
  ca : Outport  Port=2  VectorParamsAs1DForOutWhenUnconnected=off
  cb : Outport  Port=3  VectorParamsAs1DForOutWhenUnconnected=off
  stf : Outport  Port=4  VectorParamsAs1DForOutWhenUnconnected=off
  cef : Outport  Port=5  VectorParamsAs1DForOutWhenUnconnected=off
  preambleDone_upsample : Outport  Port=6  VectorParamsAs1DForOutWhenUnconnected=off
  ack : Outport  Port=7  VectorParamsAs1DForOutWhenUnconnected=off
  failed : Outport  Port=8  VectorParamsAs1DForOutWhenUnconnected=off
  valid : Outport  Port=9  VectorParamsAs1DForOutWhenUnconnected=off
  symbols : Outport  Port=10  VectorParamsAs1DForOutWhenUnconnected=off
  last : Outport  Port=11  VectorParamsAs1DForOutWhenUnconnected=off
  cumulativeCarrierPhase : Outport  Port=12  VectorParamsAs1DForOutWhenUnconnected=off
  after_cr : Outport  Port=13  VectorParamsAs1DForOutWhenUnconnected=off
  eq_ff_lms_err : Outport  Port=14  VectorParamsAs1DForOutWhenUnconnected=off
  packed_valid : Outport  Port=15  VectorParamsAs1DForOutWhenUnconnected=off
  packed_symbol : Outport  Port=16  VectorParamsAs1DForOutWhenUnconnected=off
  freeze_out : Outport  Port=17  VectorParamsAs1DForOutWhenUnconnected=off
  coarse_cfo_correct_steps : Outport  Port=18  VectorParamsAs1DForOutWhenUnconnected=off
  packed_last : Outport  Port=19  VectorParamsAs1DForOutWhenUnconnected=off
  packet_reset_feedback : Outport  Port=20
  afterTR : Outport  Port=21
  wires:
  slow_rx_baseband_outer/25(afterTR) -> afterTR/1
  slow_rx_baseband_outer/24(packet_reset_feedback) -> packet_reset_feedback/1
  agc_pwr_est/1 -> Delay3/1
  cr_p1/1 -> slow_rx_baseband_outer/7(cr_p)
  freeze_on_cef_done/1 -> slow_rx_baseband_outer/11(freeze_on_cefDone)
  slow_rx_baseband_outer/10(valid) -> valid/1
  slow_rx_baseband_outer/3(cb) -> cb/1
  slow_rx_baseband_outer/12(last) -> last/1
  slow_rx_baseband_outer/21(packed_symbol) -> packed_symbol/1
  slow_rx_baseband_outer/22(packed_last) -> packed_last/1
  freeze_en_cr_phase/1 -> slow_rx_baseband_outer/14(phase_freeze_en_cr)
  cr_i1/1 -> slow_rx_baseband_outer/8(cr_i)
  freeze_on_stf_done/1 -> slow_rx_baseband_outer/10(freeze_on_stfDone)
  slow_rx_baseband_outer/4(cb_pos) -> Terminator9/1
  data_in/1 -> Delay2/1
  slow_rx_baseband_outer/11(symbols) -> symbols/1
  slow_rx_baseband_outer/5(stf) -> stf/1
  slow_rx_baseband_outer/19(coarse_cfo_correct_steps) -> coarse_cfo_correct_steps/1
  slow_rx_baseband_outer/23(packed_err) -> Terminator1/1
  slow_rx_baseband_outer/9(failed) -> failed/1
  slow_rx_baseband_outer/16(after_cr) -> after_cr/1
  slow_rx_baseband_outer/15(carrier_phase_correction) -> cumulativeCarrierPhase/1
  slow_rx_baseband_outer/1(ca_pos) -> Terminator10/1
  slow_rx_baseband_outer/14(carrier_phase_filtered) -> Terminator7/1
  slow_rx_baseband_outer/18(eq_ff_lms_err) -> eq_ff_lms_err/1
  freeze_en_cr_int2/1 -> slow_rx_baseband_outer/13(int2_freeze_en_cr)
  slow_rx_baseband_outer/13(carrier_phase_offset) -> Terminator8/1
  slow_rx_baseband_outer/17(freeze) -> freeze_out/1
  freeze_en_cr_int1/1 -> slow_rx_baseband_outer/15(int1_freeze_en_cr)
  cr_sat2_low/1 -> slow_rx_baseband_outer/19(cr_sat2_low)
  slow_rx_baseband_outer/8(ack) -> ack/1
  slow_rx_baseband_outer/20(packed_valid) -> packed_valid/1
  cr_int1_sat_up/1 -> slow_rx_baseband_outer/16(cr_int1_sat_up)
  post_cr_i_offset/1 -> slow_rx_baseband_outer/4(post_cr_i_offset)
  eq_step/1 -> slow_rx_baseband_outer/20(eq_step)
  post_cr_q_offset/1 -> slow_rx_baseband_outer/5(post_cr_q_offset)
  cr_integrator1_decay1/1 -> slow_rx_baseband_outer/9(cr_integrator1_decay)
  cr_sat2_up/1 -> slow_rx_baseband_outer/18(cr_sat2_up)
  slow_rx_baseband_outer/2(ca) -> ca/1
  cr_i_preamp1/1 -> slow_rx_baseband_outer/6(cr_i_preamp)
  freeze_on_valid/1 -> slow_rx_baseband_outer/12(freeze_on_valid)
  enb/1 -> Delay4/1
  cr_int1_sat_low/1 -> slow_rx_baseband_outer/17(cr_int1_sat_low)
  slow_rx_baseband_outer/6(cef) -> cef/1
  slow_rx_baseband_outer/7(preamble_done) -> preambleDone_upsample/1
  eq_step_meta/1 -> slow_rx_baseband_outer/21(eq_step_meta)
  Delay2/1 -> slow_rx_baseband_outer/1(Data_In)
  Delay3/1 -> slow_rx_baseband_outer/2(agc_pwr_est)
  Delay4/1 -> strobe/1, slow_rx_baseband_outer/3(enb)

== system cyclopsLib/cyclops_rx_combined/fast_rx/fast_rx_baseband_encapsulated/fast_rx_baseband ==
  sig_in_i : Inport
  sig_in_q : Inport  Port=2
  timing_p : Inport  Port=3
  packet_reset_feedback : Inport  Port=4
  Complex to Real-Imag : ComplexToRealImag
  Real-Imag to Complex : RealImagToComplex
  Timing Recovery : Subsystem
  pipeline_delay{1..2,4,10} (4 alike) : Delay  DelayLength=regular_pipeline
  push : Outport  VectorParamsAs1DForOutWhenUnconnected=off
  data_out : Outport  Port=2  VectorParamsAs1DForOutWhenUnconnected=off
  timing_delay : Outport  Port=3  VectorParamsAs1DForOutWhenUnconnected=off
  after_agc_I : Outport  Port=4  VectorParamsAs1DForOutWhenUnconnected=off
  after_agc_Q : Outport  Port=5  VectorParamsAs1DForOutWhenUnconnected=off
  wires:
  packet_reset_feedback/1 -> Timing Recovery/3(packet_reset_feedback)
  Timing Recovery/3(full_timing_delay) -> timing_delay/1
  Timing Recovery/1(corrected_oversampled) -> pipeline_delay1/1
  Timing Recovery/2(symbol_clock) -> pipeline_delay2/1
  pipeline_delay1/1 -> data_out/1
  pipeline_delay2/1 -> push/1
  Complex to Real-Imag/1 -> after_agc_I/1
  Complex to Real-Imag/2 -> after_agc_Q/1
  pipeline_delay4/1 -> Complex to Real-Imag/1, Timing Recovery/1(uncorrected_oversampled)
  timing_p/1 -> pipeline_delay10/1
  pipeline_delay10/1 -> Timing Recovery/2(timing_p)
  Real-Imag to Complex/1 -> pipeline_delay4/1
  sig_in_i/1 -> Real-Imag to Complex/1
  sig_in_q/1 -> Real-Imag to Complex/2

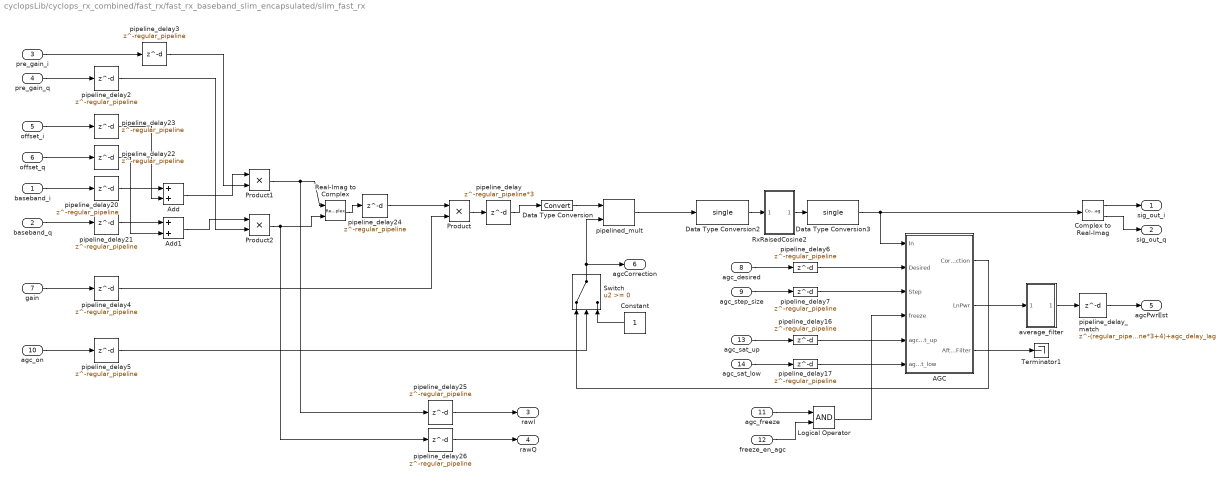
== system cyclopsLib/cyclops_rx_combined/fast_rx/fast_rx_baseband_slim_encapsulated/slim_fast_rx ==
  baseband_i : Inport
  baseband_q : Inport  Port=2
  pre_gain_i : Inport  Port=3
  pre_gain_q : Inport  Port=4
  offset_i : Inport  Port=5
  offset_q : Inport  Port=6
  gain : Inport  Port=7
  agc_desired : Inport  Port=8
  agc_step_size : Inport  Port=9
  agc_on : Inport  Port=10  OutDataTypeStr=boolean
  agc_freeze : Inport  Port=11  OutDataTypeStr=boolean
  freeze_en_agc : Inport  Port=12  OutDataTypeStr=boolean
  agc_sat_up : Inport  Port=13
  agc_sat_low : Inport  Port=14
  AGC : Subsystem  TreatAsAtomicUnit=on
  Add : Sum
  Add1 : Sum
  Complex to Real-Imag : ComplexToRealImag
  Constant : Constant  OutDataTypeStr=Inherit: Inherit via back propagation  SampleTime=-1
  Data Type Conversion : DataTypeConversion
  Data Type Conversion2 : DataTypeConversion  OutDataTypeStr=single
  Data Type Conversion3 : DataTypeConversion  OutDataTypeStr=single
  Logical Operator : Logic  AllPortsSameDT=off  OutDataTypeStr=boolean
  Product : Product  OutDataTypeStr=Inherit: Same as first input
  Product1 : Product  OutDataTypeStr=Inherit: Same as first input
  Product2 : Product  OutDataTypeStr=Inherit: Same as first input
  Real-Imag to Complex : RealImagToComplex
  RxRaisedCosine2 : Subsystem  TreatAsAtomicUnit=on
  Switch : Switch
  Terminator1 : Terminator
  average_filter : Subsystem  AncestorBlock=helperLib/average_filter  mask{pipe=regular_pipeline, samples=agcPwrAvgNum, gain=1/agcPwrAvgNum}
      mask prompts: pipe "Pipeline Delay"; samples "Samples to Average Over"; gain "Gain to Multiply Each Sample By"
  pipeline_delay : Delay  DelayLength=regular_pipeline*3
  pipeline_delay{2..7,16..17,20..26} (15 alike) : Delay  DelayLength=regular_pipeline
  pipeline_delay_match : Delay  DelayLength=(regular_pipeline*12+mult_pipeline*3+4)+agc_delay_lag
  pipelined_mult : helperLib/pipelined_mult  d=wide_mult_pipeline
  sig_out_i : Outport  VectorParamsAs1DForOutWhenUnconnected=off
  sig_out_q : Outport  Port=2  VectorParamsAs1DForOutWhenUnconnected=off
  rawI : Outport  Port=3  VectorParamsAs1DForOutWhenUnconnected=off
  rawQ : Outport  Port=4  VectorParamsAs1DForOutWhenUnconnected=off
  agcPwrEst : Outport  Port=5  VectorParamsAs1DForOutWhenUnconnected=off
  agcCorrection : Outport  Port=6  VectorParamsAs1DForOutWhenUnconnected=off
  wires:
  agc_on/1 -> pipeline_delay5/1
  Add/1 -> Product1/1
  pipeline_delay16/1 -> AGC/5(agc_sat_up)
  agc_sat_low/1 -> pipeline_delay17/1
  Data Type Conversion/1 -> pipelined_mult/1
  Switch/1 -> agcCorrection/1, pipelined_mult/2
  pipeline_delay4/1 -> Product/2
  gain/1 -> pipeline_delay4/1
  pre_gain_q/1 -> pipeline_delay2/1
  pre_gain_i/1 -> pipeline_delay3/1
  pipeline_delay20/1 -> Add/1
  Logical Operator/1 -> AGC/4(freeze)
  Real-Imag to Complex/1 -> pipeline_delay24/1
  pipeline_delay17/1 -> AGC/6(agc_sat_low)
  Add1/1 -> Product2/1
  agc_sat_up/1 -> pipeline_delay16/1
  pipeline_delay25/1 -> rawI/1
  agc_step_size/1 -> pipeline_delay7/1
  baseband_i/1 -> pipeline_delay20/1
  Product1/1 -> Real-Imag to Complex/1, pipeline_delay25/1
  pipeline_delay23/1 -> Add/2
  baseband_q/1 -> pipeline_delay21/1
  agc_desired/1 -> pipeline_delay6/1
  pipeline_delay6/1 -> AGC/2(Desired)
  pipeline_delay7/1 -> AGC/3(Step)
  Product2/1 -> Real-Imag to Complex/2, pipeline_delay26/1
  AGC/1(Correction) -> Switch/1
  pipeline_delay5/1 -> Switch/2
  pipeline_delay26/1 -> rawQ/1
  Constant/1 -> Switch/3
  AGC/2(LnPwr) -> average_filter/1(In1)
  pipeline_delay/1 -> Data Type Conversion/1
  pipeline_delay21/1 -> Add1/1
  freeze_en_agc/1 -> Logical Operator/2
  offset_q/1 -> pipeline_delay22/1
  pipeline_delay22/1 -> Add1/2
  pipeline_delay24/1 -> Product/1
  Product/1 -> pipeline_delay/1
  Data Type Conversion2/1 -> RxRaisedCosine2/1(In2)
  offset_i/1 -> pipeline_delay23/1
  average_filter/1(Out1) -> pipeline_delay_match/1
  Complex to Real-Imag/1 -> sig_out_i/1
  Complex to Real-Imag/2 -> sig_out_q/1
  pipeline_delay_match/1 -> agcPwrEst/1
  pipeline_delay2/1 -> Product2/2
  pipeline_delay3/1 -> Product1/2
  RxRaisedCosine2/1(Out2) -> Data Type Conversion3/1
  Data Type Conversion3/1 -> Complex to Real-Imag/1, AGC/1(In)
  AGC/3(AfterFilter) -> Terminator1/1
  agc_freeze/1 -> Logical Operator/1
  pipelined_mult/1 -> Data Type Conversion2/1
